simulink model "QuadControl_TrajectoryControl_I"  (R2013a)
settings: Solver=ode45  StartTime=0.0  StopTime=40  RelTol=1e-3
undefined symbols (not defined in the file or in its folder): attitudeControl, diffFlat_ur, diffFlat_xr, drawQuad, P, TrajControlI_diffFlatness, trajectory
settings Model: Creator=Raj  LastModifiedBy=raj

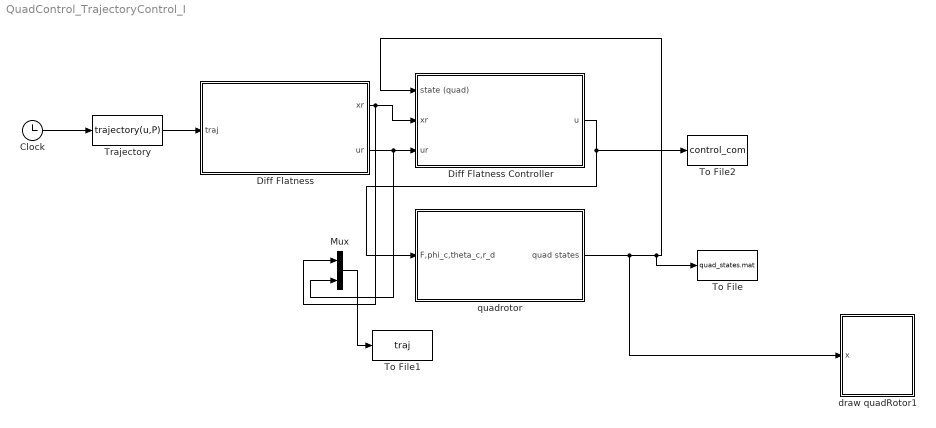
== system QuadControl_TrajectoryControl_I ==
  Clock : Clock
      settings: Decimation=100
  Diff Flatness : Subsystem
  Diff Flatness Controller : Subsystem
  Mux : Mux  Inputs=2
  To File : ToFile  Filename=quad_states.mat  MatrixName=X  SaveFormat=Timeseries
  To File1 : ToFile  Filename=traj  MatrixName=Xt  SaveFormat=Timeseries
  To File2 : ToFile  Filename=control_com  MatrixName=uc  SaveFormat=Timeseries
  Trajectory : MATLABFcn  MATLABFcn=trajectory(u,P)  OutputDimensions=12
  draw quadRotor1 : Subsystem
      mask init:
      | P.courselength = 11;
      | P.coursewidth = 6;
      |     %6ft columns plus four feet of head room
      | P.courseheight = 10;
      | 
      | % quadrotor starting point at 3 ft high and 3 ft in front of the pillars 
      | P.zstart = 0;
      | P.xstart = 0;
      | P.ystart = 0;
      | 
      | % quadrotor dimentions
      |     %2 inches from the center
      | P.boxlength = 1/6;
      | P.boxwidth = P.boxlength;
      |     %4.5 inches from the bottom to the top
      | P.boxheight = 0.375;
      |     %6 inches from box to motor
      | P.armlength = 0.5;
      |     %1/8 inch from center to the side of a rod
      | P.armwidth = 1/96;
      |     %1/4 inch from the top of the box
      | P.armposition = 1/48;
      |     %25*(2)^(1/2)/2 inches from center to perimeter along x and y axis
      | P.perimeter = 1.47;
      |     %perimeter has 3/16 inch width
      | P.periwidth = 1/64;
      | 
      | % pillar dimentions
      |     %6 ft high
      | P.pillarheight = 6;
      |     %5 ft offset;
      | P.pillarposition = 5; 
      |     %5 in radius
      | P.pillarradius = 0.417;
      |     %The adjustment for the none circular pillar
      | P.pillaradd = 0.167;
      |     %The height of each strip on color
      | P.pillarc1 = 0.833; 
      | P.pillarc2 = 0.5;
  quadrotor : Subsystem
  wires:
  Clock/1 -> Trajectory/1
  Trajectory/1 -> Diff Flatness/1(traj)
  Diff Flatness Controller/1(u) -> To File2/1, quadrotor/1(F,phi_c,theta_c,r_d)
  Diff Flatness/1(xr) -> Mux/1, Diff Flatness Controller/2("xr ")
  Diff Flatness/2(ur) -> Mux/2, Diff Flatness Controller/3(ur)
  quadrotor/1(quad states) -> draw quadRotor1/1(x), To File/1, Diff Flatness Controller/1(state (quad))
  Mux/1 -> To File1/1

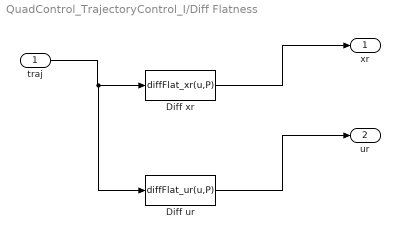
== system QuadControl_TrajectoryControl_I/Diff Flatness ==
  traj : Inport
  Diff ur : MATLABFcn  MATLABFcn=diffFlat_ur(u,P)  OutputDimensions=4
  Diff xr : MATLABFcn  MATLABFcn=diffFlat_xr(u,P)  OutputDimensions=7
  xr : Outport
  ur : Outport  Port=2
  wires:
  Diff xr/1 -> xr/1
  Diff ur/1 -> ur/1
  traj/1 -> Diff ur/1, Diff xr/1

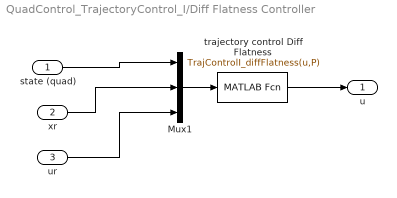
== system QuadControl_TrajectoryControl_I/Diff Flatness Controller ==
  state (quad) : Inport
  "xr " : Inport  Port=2
  ur : Inport  Port=3
  Mux1 : Mux  Inputs=3
  trajectory control Diff Flatness : MATLABFcn  MATLABFcn=TrajControlI_diffFlatness(u,P)  OutputDimensions=4
  u : Outport
  wires:
  state (quad)/1 -> Mux1/1
  Mux1/1 -> trajectory control Diff Flatness/1
  ur/1 -> Mux1/3
  "xr "/1 -> Mux1/2
  trajectory control Diff Flatness/1 -> u/1

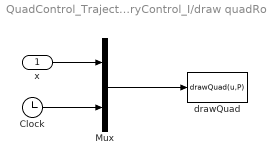
== system QuadControl_TrajectoryControl_I/draw quadRotor1 ==
  x : Inport
  Clock : Clock
  Mux : Mux  Inputs=2
  drawQuad : MATLABFcn  MATLABFcn=drawQuad(u,P)  OutputDimensions=0
  wires:
  Mux/1 -> drawQuad/1
  x/1 -> Mux/1
  Clock/1 -> Mux/2

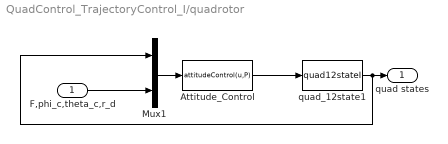
== system QuadControl_TrajectoryControl_I/quadrotor ==
  F,phi_c,theta_c,r_d : Inport
  Attitude_Control : MATLABFcn  MATLABFcn=attitudeControl(u,P)  OutputDimensions=4
  Mux1 : Mux  Inputs=2
  quad_12state1 : S-Function  FunctionName=quad12stateI  Parameters=P  EnableBusSupport=off
  quad states : Outport
  wires:
  quad_12state1/1 -> Mux1/1, quad states/1
  Attitude_Control/1 -> quad_12state1/1
  Mux1/1 -> Attitude_Control/1
  F,phi_c,theta_c,r_d/1 -> Mux1/2
